simulink model "euler_transform_pipelined"  (R2018b)
settings: Solver=FixedStepDiscrete  StartTime=0.0  StopTime=1000+3*(nIters+3)  FixedStep=1  RelTol=1e-3
undefined symbols (not defined in the file or in its folder): nIters, uIn
settings Model: DataTypeOverride=Off  Creator=jimjoy  LastModifiedBy=tbryan
settings DataIOCC: LimitDataPoints=on  SaveOutput=off  SaveTime=off
settings OptimizationCC: BlockReduction=off  ConditionallyExecuteInputs=off  DefaultParameterBehavior=Inlined  LifeSpan=inf
settings DebuggingCC: AlgebraicLoopMsg=error  SingleTaskRateTransMsg=error  AllowSymbolicDim=off  StrictBusMsg=ErrorOnBusTreatedAsVector  SFUnexpectedBacktrackingDiag=warning  SFNoUnconditionalDefaultTransitionDiag=warning  SFExecutionAtInitializationDiag=none
settings HardwareCC: ProdBitPerPointer=32  ProdBitPerSizeT=32  ProdBitPerPtrDiffT=32  ProdLargestAtomicFloat=None  ProdIntDivRoundTo=Undefined  ProdEndianess=Unspecified  ProdWordSize=32  ProdHWDeviceType=ASIC/FPGA->ASIC/FPGA  ProdEqTarget=off
settings SFSimCC: SimUseLocalCustomCode=off
settings RTWCC: RTWUseLocalCustomCode=off
settings CodeAppCC: StateflowObjectComments=on
settings GRTTargetCC: TargetLangStandard=C89/C90 (ANSI)  GeneratePreprocessorConditionals=Disable all
settings ConfigComp: CovScope=ReferencedModels  CovMetricSettings=dw  CovHtmlReporting=on  CovSaveCumulativeToWorkspaceVar=on  CovSaveSingleToWorkspaceVar=on  CovExternalEMLEnable=off  CovSFcnEnable=off

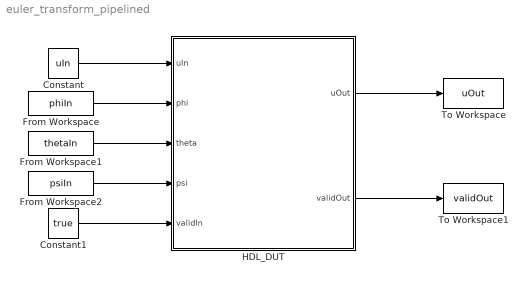
== system euler_transform_pipelined ==
  Constant : Constant  Value=uIn
  Constant1 : Constant  Value=true  SampleTime=-1
  From Workspace : FromWorkspace  VariableName=phiIn  SampleTime=1  Interpolate=off  OutputAfterFinalValue=Holding final value
  From Workspace1 : FromWorkspace  VariableName=thetaIn  SampleTime=1  Interpolate=off  OutputAfterFinalValue=Cyclic repetition
  From Workspace2 : FromWorkspace  VariableName=psiIn  SampleTime=1  Interpolate=off  OutputAfterFinalValue=Holding final value
  HDL_DUT : Subsystem
  To Workspace : ToWorkspace  VariableName=uOut  SampleTime=-1
  To Workspace1 : ToWorkspace  VariableName=validOut  SampleTime=-1
      settings: Save2DSignal=2-D array (concatenate along first dimension)
  wires:
  Constant/1 -> HDL_DUT/1(uIn)
  From Workspace/1 -> HDL_DUT/2(phi)
  From Workspace1/1 -> HDL_DUT/3(theta)
  From Workspace2/1 -> HDL_DUT/4(psi)
  Constant1/1 -> HDL_DUT/5(validIn)
  HDL_DUT/1(uOut) -> To Workspace/1
  HDL_DUT/2(validOut) -> To Workspace1/1

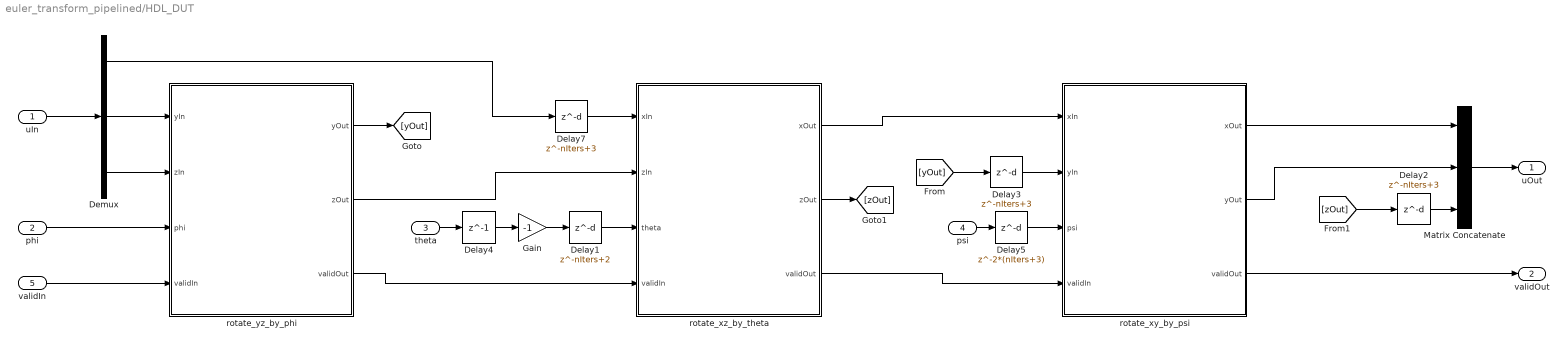
== system euler_transform_pipelined/HDL_DUT ==
  uIn : Inport
  phi : Inport  Port=2
  theta : Inport  Port=3
  psi : Inport  Port=4
  validIn : Inport  Port=5
  Delay1 : Delay  DelayLength=nIters+2
  Delay2 : Delay  DelayLength=nIters+3
  Delay3 : Delay  DelayLength=nIters+3
  Delay4 : Delay  DelayLength=1
  Delay5 : Delay  DelayLength=2*(nIters+3)
  Delay7 : Delay  DelayLength=nIters+3
  Demux : Demux  Outputs=3
  Gain : Gain  Gain=-1  OutDataTypeStr=Inherit: Same as input
  Matrix Concatenate : Concatenate  NumInputs=3  ConcatenateDimension=2
  rotate_xy_by_psi : Subsystem
  rotate_xz_by_theta : Subsystem
  rotate_yz_by_phi : Subsystem
  uOut : Outport
  validOut : Outport  Port=2
  wires:
  uIn/1 -> Demux/1
  Demux/2 -> rotate_yz_by_phi/1(yIn)
  Demux/3 -> rotate_yz_by_phi/2(zIn)
  phi/1 -> rotate_yz_by_phi/3(phi)
  validIn/1 -> rotate_yz_by_phi/4(validIn)
  Demux/1 -> Delay7/1
  rotate_yz_by_phi/2(zOut) -> rotate_xz_by_theta/2(zIn)
  rotate_yz_by_phi/3(validOut) -> rotate_xz_by_theta/4(validIn)
  Matrix Concatenate/1 -> uOut/1
  rotate_xz_by_theta/1(xOut) -> rotate_xy_by_psi/1(xIn)
  rotate_xz_by_theta/3(validOut) -> rotate_xy_by_psi/4(validIn)
  rotate_xy_by_psi/1(xOut) -> Matrix Concatenate/1
  rotate_xy_by_psi/2(yOut) -> Matrix Concatenate/2
  theta/1 -> Delay4/1
  Delay1/1 -> rotate_xz_by_theta/3(theta)
  rotate_xy_by_psi/3(validOut) -> validOut/1
  Delay2/1 -> Matrix Concatenate/3
  Delay3/1 -> rotate_xy_by_psi/2(yIn)
  Delay5/1 -> rotate_xy_by_psi/3(psi)
  Delay7/1 -> rotate_xz_by_theta/1(xIn)
  rotate_yz_by_phi/1(yOut) -> [yOut]
  psi/1 -> Delay5/1
  [yOut] -> Delay3/1
  rotate_xz_by_theta/2(zOut) -> [zOut]
  [zOut] -> Delay2/1
  Delay4/1 -> Gain/1
  Gain/1 -> Delay1/1

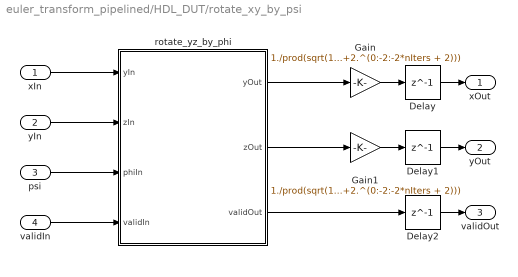
== system euler_transform_pipelined/HDL_DUT/rotate_xy_by_psi ==
  xIn : Inport
  yIn : Inport  Port=2
  psi : Inport  Port=3
  validIn : Inport  Port=4
  Delay : Delay  DelayLength=1
  Delay1 : Delay  DelayLength=1
  Delay2 : Delay  DelayLength=1
  Gain : Gain  Gain=1./prod(sqrt(1+2.^(0:-2:-2*nIters + 2)))  OutDataTypeStr=Inherit: Same as input
  Gain1 : Gain  Gain=1./prod(sqrt(1+2.^(0:-2:-2*nIters + 2)))  OutDataTypeStr=Inherit: Same as input
  rotate_yz_by_phi : MATLAB Function  TreatAsAtomicUnit=on  mask{nIters=nIters}
      mask prompts: nIters "Number of CORDIC Iterations"
  xOut : Outport
  yOut : Outport  Port=2
  validOut : Outport  Port=3
  wires:
  xIn/1 -> rotate_yz_by_phi/1(yIn)
  yIn/1 -> rotate_yz_by_phi/2(zIn)
  psi/1 -> rotate_yz_by_phi/3(phiIn)
  validIn/1 -> rotate_yz_by_phi/4(validIn)
  rotate_yz_by_phi/1(yOut) -> Gain/1
  Gain/1 -> Delay/1
  rotate_yz_by_phi/2(zOut) -> Gain1/1
  Gain1/1 -> Delay1/1
  rotate_yz_by_phi/3(validOut) -> Delay2/1
  Delay/1 -> xOut/1
  Delay1/1 -> yOut/1
  Delay2/1 -> validOut/1

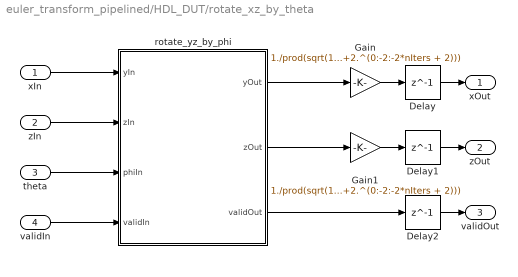
== system euler_transform_pipelined/HDL_DUT/rotate_xz_by_theta ==
  xIn : Inport
  zIn : Inport  Port=2
  theta : Inport  Port=3
  validIn : Inport  Port=4
  Delay : Delay  DelayLength=1
  Delay1 : Delay  DelayLength=1
  Delay2 : Delay  DelayLength=1
  Gain : Gain  Gain=1./prod(sqrt(1+2.^(0:-2:-2*nIters + 2)))  OutDataTypeStr=Inherit: Same as input
  Gain1 : Gain  Gain=1./prod(sqrt(1+2.^(0:-2:-2*nIters + 2)))  OutDataTypeStr=Inherit: Same as input
  rotate_yz_by_phi : MATLAB Function  TreatAsAtomicUnit=on  mask{nIters=nIters}
      mask prompts: nIters "Number of CORDIC Iterations"
  xOut : Outport
  zOut : Outport  Port=2
  validOut : Outport  Port=3
  wires:
  xIn/1 -> rotate_yz_by_phi/1(yIn)
  zIn/1 -> rotate_yz_by_phi/2(zIn)
  theta/1 -> rotate_yz_by_phi/3(phiIn)
  validIn/1 -> rotate_yz_by_phi/4(validIn)
  rotate_yz_by_phi/1(yOut) -> Gain/1
  Gain/1 -> Delay/1
  rotate_yz_by_phi/2(zOut) -> Gain1/1
  Gain1/1 -> Delay1/1
  rotate_yz_by_phi/3(validOut) -> Delay2/1
  Delay/1 -> xOut/1
  Delay1/1 -> zOut/1
  Delay2/1 -> validOut/1

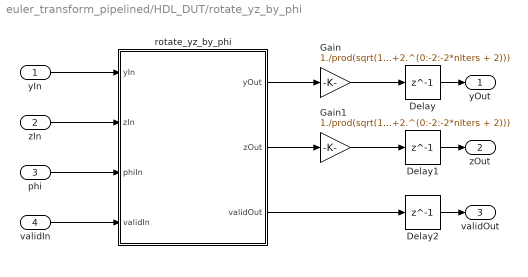
== system euler_transform_pipelined/HDL_DUT/rotate_yz_by_phi ==
  yIn : Inport
  zIn : Inport  Port=2
  phi : Inport  Port=3
  validIn : Inport  Port=4
  Delay : Delay  DelayLength=1
  Delay1 : Delay  DelayLength=1
  Delay2 : Delay  DelayLength=1
  Gain : Gain  Gain=1./prod(sqrt(1+2.^(0:-2:-2*nIters + 2)))  OutDataTypeStr=Inherit: Same as input
  Gain1 : Gain  Gain=1./prod(sqrt(1+2.^(0:-2:-2*nIters + 2)))  OutDataTypeStr=Inherit: Same as input
  rotate_yz_by_phi : MATLAB Function  TreatAsAtomicUnit=on  mask{nIters=nIters}
      mask prompts: nIters "Number of CORDIC Iterations"
  yOut : Outport
  zOut : Outport  Port=2
  validOut : Outport  Port=3
  wires:
  yIn/1 -> rotate_yz_by_phi/1(yIn)
  zIn/1 -> rotate_yz_by_phi/2(zIn)
  phi/1 -> rotate_yz_by_phi/3(phiIn)
  validIn/1 -> rotate_yz_by_phi/4(validIn)
  rotate_yz_by_phi/1(yOut) -> Gain/1
  Gain/1 -> Delay/1
  rotate_yz_by_phi/2(zOut) -> Gain1/1
  Gain1/1 -> Delay1/1
  rotate_yz_by_phi/3(validOut) -> Delay2/1
  Delay/1 -> yOut/1
  Delay1/1 -> zOut/1
  Delay2/1 -> validOut/1

== matlab function euler_transform_pipelined/HDL_DUT/rotate_xz_by_theta/rotate_yz_by_phi ==
  settings: fimath=hdlfimath
  data: yIn input; zIn input; yOut output; zOut output; phiIn input; validIn input; validOut output; nIters parameter
function [yOut, zOut, validOut] = rotate_by_phi(yIn, zIn, phiIn, validIn, nIters)
    %#codegen
    
    %Copyright 2018 The MathWorks, Inc.
    
    persistent yReg zReg validReg phiReg
    
    yNumericTypeInternal = numerictype(1,yIn.WordLength + 3, yIn.FractionLength + 3);
    zNumericTypeInternal = numerictype(1,zIn.WordLength + 3, zIn.FractionLength + 3);
    phiNumericTypeInternal = numerictype(1,zIn.WordLength+3, zIn.FractionLength + 3);
    
    if isempty(yReg)
        yReg = fi(zeros(1,nIters+2), yNumericTypeInternal);
        zReg = fi(zeros(1,nIters+2), zNumericTypeInternal);
        phiReg = fi(zeros(1,nIters+2), phiNumericTypeInternal);
        validReg = false(1,nIters+2);
    end
    
    yOut = cast(yReg(end),'like',yIn);
    zOut = cast(zReg(end),'like',zIn);
    validOut = validReg(end);
    %coder.unroll
    for ii = nIters+2:-1:3
            validReg(ii) = validReg(ii - 1);
            [yReg(ii), zReg(ii), phiReg(ii)] = ...
                cordicRotationKernel(yReg(ii-1), zReg(ii - 1), phiReg(ii - 1),...
                ii, nIters);
    end
    
    validReg(2) = validReg(1);
    [yReg(2), zReg(2), phiReg(2)] = ...
                cordicQuadrantCorrection(yReg(1), zReg(1), phiReg(1));
    
    [yReg(1), zReg(1), phiReg(1), validReg(1)] = ...
                readInputs(yIn, zIn, phiIn, validIn);
    
end

function [y, z, phi, valid] = readInputs(yIn, zIn, phiIn, validIn)
    y = yIn;
    z = zIn;
    phi = phiIn;
    valid = validIn;
end

function [yOut, zOut, phiOut] = cordicQuadrantCorrection(y, z, phi)
    yOut = y;
    zOut = z;
    phiOut = phi;
    if (phi > coder.const(cast(pi/2,'like',phi))) && ...
            (phi < coder.const(cast(1.5*pi,'like',phi)))
        phiOut(:) = phi - cast(pi,'like',phi);
        yOut(:) = -y;
        zOut(:) = -z;
    elseif (phi > coder.const(cast(1.5*pi,'like',phi)))
        phiOut(:) = phi - cast(2*pi,'like',phi);
        yOut(:) = y;
        zOut(:) = z;
    elseif (phi < coder.const(cast(-pi/2,'like',phi)))
        phiOut(:) = phi + cast(pi,'like',phi);
        yOut(:) = -y;
        zOut(:) = -z;
    else
        phiOut(:) = phi;
        yOut(:) = y;
        zOut(:) = z;
    end
end

function [yOut, zOut, phiOut] = cordicRotationKernel(y, z, phi, iterNum, numIters)
    angleTable = coder.const(getAngleTable(numIters,phi));
    y0 = bitsra(y,iterNum - 3);
    z0 = bitsra(z,iterNum - 3);
    yOut = y;
    zOut = z;
    phiOut = phi;
    if phi > 0
        % Rotate in the positive direction
        yOut(:) = y - z0;
        zOut(:) = z + y0;
        phiOut(:) = phi - angleTable(iterNum - 2);
    else
        % Rotate in the negative direction
        yOut(:) = y + z0;
        zOut(:) = z - y0;
        phiOut(:) = phi + angleTable(iterNum - 2);
    end
end

function angleTable = getAngleTable(numIters, T)
    angleTable = cast(atan(2.^(0:-1:-numIters + 1)),'like',T);
end

== matlab function euler_transform_pipelined/HDL_DUT/rotate_yz_by_phi/rotate_yz_by_phi ==
  settings: fimath=hdlfimath
  data: yIn input; zIn input; yOut output; zOut output; phiIn input; validIn input; validOut output; nIters parameter
function [yOut, zOut, validOut] = rotate_by_phi(yIn, zIn, phiIn, validIn, nIters)
    %#codegen
    
    %Copyright 2018 The MathWorks, Inc.
    
    persistent yReg zReg validReg phiReg
    
    yNumericTypeInternal = numerictype(1,yIn.WordLength + 3, yIn.FractionLength + 3);
    zNumericTypeInternal = numerictype(1,zIn.WordLength + 3, zIn.FractionLength + 3);
    phiNumericTypeInternal = numerictype(1,zIn.WordLength+3, zIn.FractionLength + 3);
    
    if isempty(yReg)
        yReg = fi(zeros(1,nIters+2), yNumericTypeInternal);
        zReg = fi(zeros(1,nIters+2), zNumericTypeInternal);
        phiReg = fi(zeros(1,nIters+2), phiNumericTypeInternal);
        validReg = false(1,nIters+2);
    end
    
    yOut = cast(yReg(end),'like',yIn);
    zOut = cast(zReg(end),'like',zIn);
    validOut = validReg(end);
    %coder.unroll
    for ii = nIters+2:-1:3
            validReg(ii) = validReg(ii - 1);
            [yReg(ii), zReg(ii), phiReg(ii)] = ...
                cordicRotationKernel(yReg(ii-1), zReg(ii - 1), phiReg(ii - 1),...
                ii, nIters);
    end
    
    validReg(2) = validReg(1);
            [yReg(2), zReg(2), phiReg(2)] = ...
                cordicQuadrantCorrection(yReg(1), zReg(1), phiReg(1));
    
    [yReg(1), zReg(1), phiReg(1), validReg(1)] = ...
                readInputs(yIn, zIn, phiIn, validIn);
    
end

function [y, z, phi, valid] = readInputs(yIn, zIn, phiIn, validIn)
    y = yIn;
    z = zIn;
    phi = phiIn;
    valid = validIn;
end

function [yOut, zOut, phiOut] = cordicQuadrantCorrection(y, z, phi)
    yOut = y;
    zOut = z;
    phiOut = phi;
    if (phi > coder.const(cast(pi/2,'like',phi))) && ...
            (phi < coder.const(cast(1.5*pi,'like',phi)))
        phiOut(:) = phi - cast(pi,'like',phi);
        yOut(:) = -y;
        zOut(:) = -z;
    elseif (phi > coder.const(cast(1.5*pi,'like',phi)))
        phiOut(:) = phi - cast(2*pi,'like',phi);
        yOut(:) = y;
        zOut(:) = z;
    end
end

function [yOut, zOut, phiOut] = cordicRotationKernel(y, z, phi, iterNum, numIters)
    angleTable = coder.const(getAngleTable(numIters,phi));
    y0 = bitsra(y,iterNum - 3);
    z0 = bitsra(z,iterNum - 3);
    yOut = y;
    zOut = z;
    phiOut = phi;
    if phi > 0
        % Rotate in the positive direction
        yOut(:) = y - z0;
        zOut(:) = z + y0;
        phiOut(:) = phi - angleTable(iterNum - 2);
    else
        % Rotate in the negative direction
        yOut(:) = y + z0;
        zOut(:) = z - y0;
        phiOut(:) = phi + angleTable(iterNum - 2);
    end
end

function angleTable = getAngleTable(numIters, T)
    angleTable = cast(atan(2.^(0:-1:-numIters + 1)),'like',T);
end

== matlab function euler_transform_pipelined/HDL_DUT/rotate_xy_by_psi/rotate_yz_by_phi ==
  settings: fimath=hdlfimath
  data: yIn input; zIn input; yOut output; zOut output; phiIn input; validIn input; validOut output; nIters parameter
function [yOut, zOut, validOut] = rotate_by_phi(yIn, zIn, phiIn, validIn, nIters)
    %#codegen
    
    %Copyright 2018 The MathWorks, Inc.
    
    persistent yReg zReg validReg phiReg
    
    yNumericTypeInternal = numerictype(1,yIn.WordLength + 3, yIn.FractionLength + 3);
    zNumericTypeInternal = numerictype(1,zIn.WordLength + 3, zIn.FractionLength + 3);
    phiNumericTypeInternal = numerictype(1,zIn.WordLength+3, zIn.FractionLength + 3);
    
    if isempty(yReg)
        yReg = fi(zeros(1,nIters+2), yNumericTypeInternal);
        zReg = fi(zeros(1,nIters+2), zNumericTypeInternal);
        phiReg = fi(zeros(1,nIters+2), phiNumericTypeInternal);
        validReg = false(1,nIters+2);
    end
    
    yOut = cast(yReg(end),'like',yIn);
    zOut = cast(zReg(end),'like',zIn);
    validOut = validReg(end);
    %coder.unroll
    for ii = nIters+2:-1:3
            validReg(ii) = validReg(ii - 1);
            [yReg(ii), zReg(ii), phiReg(ii)] = ...
                cordicRotationKernel(yReg(ii-1), zReg(ii - 1), phiReg(ii - 1),...
                ii, nIters);
    end
    
    validReg(2) = validReg(1);
            [yReg(2), zReg(2), phiReg(2)] = ...
                cordicQuadrantCorrection(yReg(1), zReg(1), phiReg(1));
    
    [yReg(1), zReg(1), phiReg(1), validReg(1)] = ...
                readInputs(yIn, zIn, phiIn, validIn);
    
end

function [y, z, phi, valid] = readInputs(yIn, zIn, phiIn, validIn)
    y = yIn;
    z = zIn;
    phi = phiIn;
    valid = validIn;
end

function [yOut, zOut, phiOut] = cordicQuadrantCorrection(y, z, phi)
    yOut = y;
    zOut = z;
    phiOut = phi;
    if (phi > coder.const(cast(pi/2,'like',phi))) && ...
            (phi < coder.const(cast(1.5*pi,'like',phi)))
        phiOut(:) = phi - cast(pi,'like',phi);
        yOut(:) = -y;
        zOut(:) = -z;
    elseif (phi > coder.const(cast(1.5*pi,'like',phi)))
        phiOut(:) = phi - cast(2*pi,'like',phi);
        yOut(:) = y;
        zOut(:) = z;
    end
end

function [yOut, zOut, phiOut] = cordicRotationKernel(y, z, phi, iterNum, numIters)
    angleTable = coder.const(getAngleTable(numIters,phi));
    y0 = bitsra(y,iterNum - 3);
    z0 = bitsra(z,iterNum - 3);
    yOut = y;
    zOut = z;
    phiOut = phi;
    if phi > 0
        % Rotate in the positive direction
        yOut(:) = y - z0;
        zOut(:) = z + y0;
        phiOut(:) = phi - angleTable(iterNum - 2);
    else
        % Rotate in the negative direction
        yOut(:) = y + z0;
        zOut(:) = z - y0;
        phiOut(:) = phi + angleTable(iterNum - 2);
    end
end

function angleTable = getAngleTable(numIters, T)
    angleTable = cast(atan(2.^(0:-1:-numIters + 1)),'like',T);
end
